simulink model "model_problem9"  (R2020a)
settings: Solver=VariableStepAuto  StartTime=0.0  StopTime=10.0  RelTol=1e-3
undefined symbols (not defined in the file): Kd, Ki, Kp
settings Model: Creator=Prateek  LastModifiedBy=Prateek

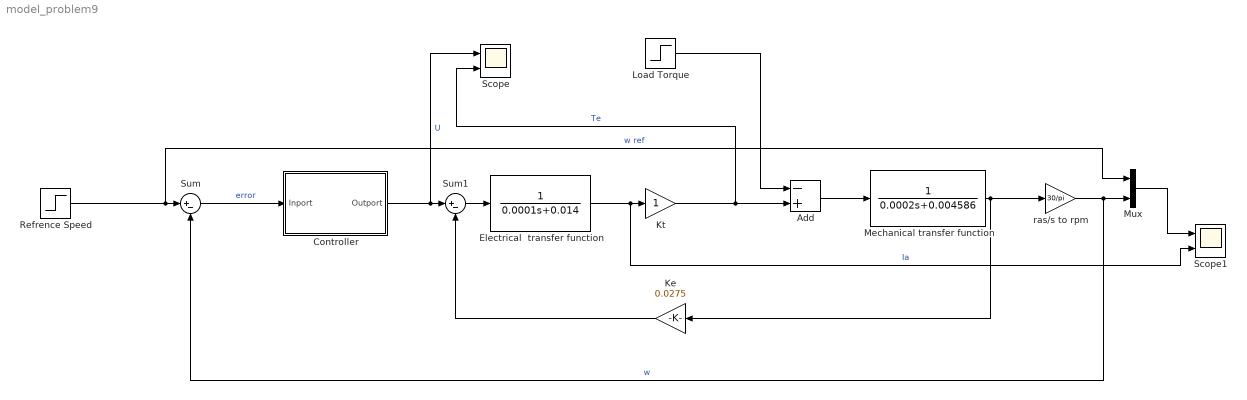
== system model_problem9 ==
  Add : Sum  Inputs=-+
  Controller : Subsystem
  Electrical  transfer function : TransferFcn  Denominator=[0.0001 0.014]
  Ke : Gain  Gain=0.0275
  Kt : Gain
  Load Torque : Step  Time=0.1  After=10  SampleTime=0
  Mechanical transfer function : TransferFcn  Denominator=[0.0002 0.004586]
  Mux : Mux  Inputs=2
  Refrence Speed : Step  After=1500  SampleTime=0
  Scope : Scope  NumInputPorts=2
  Scope1 : Scope  NumInputPorts=2
  Sum : Sum  Inputs=|+-
  Sum1 : Sum  Inputs=|+-
  ras/s to rpm : Gain  Gain=30/pi
  wires:
  Refrence Speed/1 -> Mux/1, Sum/1  "w ref"
  Sum/1 -> Controller/1(Inport)  "error"
  Controller/1(Outport) -> Scope/1, Sum1/1  "U"
  Sum1/1 -> Electrical  transfer function/1
  Electrical  transfer function/1 -> Scope1/2, Kt/1  "Ia"
  Load Torque/1 -> Add/1
  Kt/1 -> Scope/2, Add/2  "Te"
  Add/1 -> Mechanical transfer function/1
  Mux/1 -> Scope1/1
  Mechanical transfer function/1 -> Ke/1, ras/s to rpm/1
  Ke/1 -> Sum1/2
  ras/s to rpm/1 -> Sum/2, Mux/2  "w"

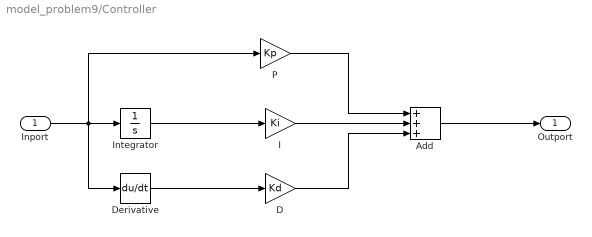
== system model_problem9/Controller ==
  Inport : Inport
  Add : Sum  Inputs=+++
  D : Gain  Gain=Kd
  Derivative : Derivative
  I : Gain  Gain=Ki
  Integrator : Integrator
  P : Gain  Gain=Kp
  Outport : Outport
  wires:
  Inport/1 -> P/1, Integrator/1, Derivative/1
  D/1 -> Add/3
  P/1 -> Add/1
  I/1 -> Add/2
  Add/1 -> Outport/1
  Integrator/1 -> I/1
  Derivative/1 -> D/1
